simulink model "modeling"  (R2023b)
settings: Solver=VariableStepAuto  StartTime=0.0  StopTime=10.0  RelTol=1e-3
undefined symbols (not defined in the file or in its folder): k_values, y
settings Model: Creator=Катя  LastModifiedBy=Катя

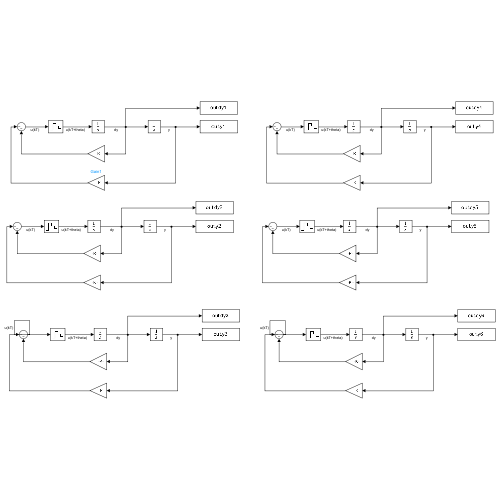
[thumbnail: Simulink's stored preview of the top-level diagram]
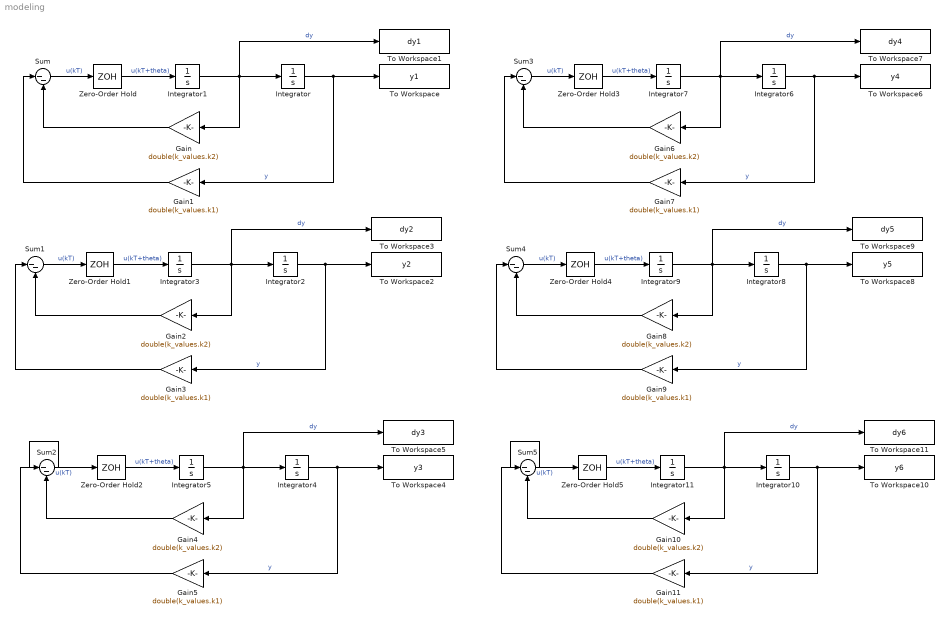
== system modeling ==
  Gain{,2,4,6,8,10} (6 alike) : Gain  Gain=double(k_values.k2)
  Gain{1,3,5,7,9,11} (6 alike) : Gain  Gain=double(k_values.k1)
  Integrator : Integrator  InitialCondition=y(1)
  Integrator{1,3,5,7,9,11} (6 alike) : Integrator
  Integrator10 : Integrator  InitialCondition=y(6)
  Integrator2 : Integrator  InitialCondition=y(2)
  Integrator4 : Integrator  InitialCondition=y(3)
  Integrator6 : Integrator  InitialCondition=y(4)
  Integrator8 : Integrator  InitialCondition=y(5)
  Sum{,1..5} (6 alike) : Sum  Inputs=|--
  To Workspace : ToWorkspace  VariableName=y1  SaveFormat=Timeseries  SampleTime=-1
  To Workspace1 : ToWorkspace  VariableName=dy1  SaveFormat=Timeseries  SampleTime=-1
  To Workspace10 : ToWorkspace  VariableName=y6  SaveFormat=Timeseries  SampleTime=-1
  To Workspace11 : ToWorkspace  VariableName=dy6  SaveFormat=Timeseries  SampleTime=-1
  To Workspace2 : ToWorkspace  VariableName=y2  SaveFormat=Timeseries  SampleTime=-1
  To Workspace3 : ToWorkspace  VariableName=dy2  SaveFormat=Timeseries  SampleTime=-1
  To Workspace4 : ToWorkspace  VariableName=y3  SaveFormat=Timeseries  SampleTime=-1
  To Workspace5 : ToWorkspace  VariableName=dy3  SaveFormat=Timeseries  SampleTime=-1
  To Workspace6 : ToWorkspace  VariableName=y4  SaveFormat=Timeseries  SampleTime=-1
  To Workspace7 : ToWorkspace  VariableName=dy4  SaveFormat=Timeseries  SampleTime=-1
  To Workspace8 : ToWorkspace  VariableName=y5  SaveFormat=Timeseries  SampleTime=-1
  To Workspace9 : ToWorkspace  VariableName=dy5  SaveFormat=Timeseries  SampleTime=-1
  Zero-Order Hold{,1..5} (6 alike) : ZeroOrderHold  SampleTime=-1
  wires:
  Integrator1/1 -> To Workspace1/1, Gain/1, Integrator/1  "dy"
  Zero-Order Hold/1 -> Integrator1/1  "u(kT+theta)"
  Integrator/1 -> To Workspace/1, Gain1/1  "y"
  Sum/1 -> Zero-Order Hold/1  "u(kT)"
  Gain/1 -> Sum/2
  Gain1/1 -> Sum/1
  Gain3/1 -> Sum1/1
  Integrator2/1 -> To Workspace2/1, Gain3/1  "y"
  Zero-Order Hold1/1 -> Integrator3/1  "u(kT+theta)"
  Gain2/1 -> Sum1/2
  Integrator3/1 -> To Workspace3/1, Gain2/1, Integrator2/1  "dy"
  Sum1/1 -> Zero-Order Hold1/1  "u(kT)"
  Zero-Order Hold2/1 -> Integrator5/1  "u(kT+theta)"
  Gain5/1 -> Sum2/1
  Integrator4/1 -> To Workspace4/1, Gain5/1  "y"
  Gain4/1 -> Sum2/2
  Sum2/1 -> Zero-Order Hold2/1  "u(kT)"
  Integrator5/1 -> To Workspace5/1, Gain4/1, Integrator4/1  "dy"
  Integrator11/1 -> To Workspace11/1, Gain10/1, Integrator10/1  "dy"
  Integrator10/1 -> To Workspace10/1, Gain11/1  "y"
  Gain10/1 -> Sum5/2
  Zero-Order Hold5/1 -> Integrator11/1  "u(kT+theta)"
  Sum3/1 -> Zero-Order Hold3/1  "u(kT)"
  Zero-Order Hold3/1 -> Integrator7/1  "u(kT+theta)"
  Sum5/1 -> Zero-Order Hold5/1  "u(kT)"
  Integrator6/1 -> To Workspace6/1, Gain7/1  "y"
  Gain6/1 -> Sum3/2
  Gain9/1 -> Sum4/1
  Integrator8/1 -> To Workspace8/1, Gain9/1  "y"
  Gain8/1 -> Sum4/2
  Gain7/1 -> Sum3/1
  Sum4/1 -> Zero-Order Hold4/1  "u(kT)"
  Gain11/1 -> Sum5/1
  Integrator7/1 -> To Workspace7/1, Gain6/1, Integrator6/1  "dy"
  Zero-Order Hold4/1 -> Integrator9/1  "u(kT+theta)"
  Integrator9/1 -> To Workspace9/1, Gain8/1, Integrator8/1  "dy"
